simulink model "MPC_framework"  (Simulink 6.4)
settings: Solver=FixedStepDiscrete  StartTime=0.0  StopTime=10.0  FixedStep=0.01  RelTol=1e-3
PreLoadFcn:
  | RTWConfigurationCB('preloadfcn', bdroot);
InitFcn:
  | % START RTW CONFIGURATION CODE %
  | RTWConfigurationCB('rtw_target_initfcn',gcs);
  | % END RTW CONFIGURATION CODE %
undefined symbols (not defined in the file): a1, a2, DA_max_saturation, DA_min_saturation, DiscIntNeverNeededParam, fundamental_sample_time, incntr_half_val, init_1_message, init_2_message, init_ack_async_message, init_ack_sync_message, motor_negative_value_seg_1, motor_negative_value_seg_2, motor_positive_value_seg_1, motor_positive_value_seg_2, motor_stopped_value, ticks_per_trajectory_time, trajectory_time
libraries: canblocks x16, mpc555toucan x16, simulink x8, mpc555drivers x1
(part 2 of 2)

== stateflow chart State Machine ==
  settings: updateMethod=DISCRETE  sampleTime=0.01  executeAtInitialization=1
  state INIT
    entry: init_out_value=init_1_message;
    init_out_enable=1;
  state INIT_ACK
    entry: init_out_enable=0;
    init_out_value=init_2_message;
    init_out_trigger=1;
  state OPERATION
    entry: operation_mode=255;
    controller_enable=0;
    trajectory_enable=0;
    state PRIMITIVE
      entry: operation_mode=1;
      during: controller_enable=0;
      exit: motor1_reference=motor_stopped_value;
      motor2_reference=motor_stopped_value;
      state STOPPED
        entry: motor1_reference=motor_stopped_value;
        motor2_reference=motor_stopped_value;
        da_out_trigger=1;
        during: motor1_reference=motor_stopped_value;
        motor2_reference=motor_stopped_value;
        da_out_trigger=1;
        exit: stop_trigger=0;
      state MOVING
        state POSITIVE_MOV_SEG_1
          entry: motor2_reference=motor_stopped_value;
          during:
          motor1_reference=motor_positive_value_seg_1;
          da_out_trigger=1;
        state NEGATIVE_MOV_SEG_1
          entry: motor2_reference=motor_stopped_value;
          during:
          motor1_reference=motor_negative_value_seg_1;
          da_out_trigger=1;
        state POSITIVE_MOV_SEG_2
          entry: motor1_reference=motor_stopped_value;
          during:
          motor2_reference=motor_positive_value_seg_2;
          da_out_trigger=1;
        state NEGATIVE_MOV_SEG_2
          entry: motor1_reference=motor_stopped_value;
          during:
          motor2_reference=motor_negative_value_seg_2;
          da_out_trigger=1;
      (default) -> STOPPED
      MOVING -> STOPPED : [primitive_button==5]
      STOPPED -> POSITIVE_MOV_SEG_1 [order 4] : [primitive_button==1]
      STOPPED -> NEGATIVE_MOV_SEG_1 [order 2] : [primitive_button==3]
      STOPPED -> POSITIVE_MOV_SEG_2 [order 3] : [primitive_button==2]
      STOPPED -> NEGATIVE_MOV_SEG_2 [order 1] : [primitive_button==4]
    state CONTROLLER
      entry: operation_mode=2;
      alpha1_ref=alpha_in[0];
      alpha2_ref=alpha_in[1];
      motor1_reference=alpha1_ref;
      motor2_reference=alpha2_ref;
      trajectory_enable=0;
      controller_enable=1;
      da_out_trigger=1;
      exit: motor1_reference=motor_stopped_value;
      motor2_reference=motor_stopped_value;
      state HOLD
        entry:
        trajectory_ready=0;
        controller_message=4;
        send_controller_message;
        state HOLD_main
        state HOLD_wait
        (default) -> HOLD_main
        HOLD_main -> (junction 20) : [invgeo_done==1]
        (junction 21) -> HOLD_main : /send_controller_message
        (junction 20) -> (junction 23) [order 1] : [invgeo_error==0]{controller_message=1}
        (junction 20) -> (junction 24) [order 2] : [invgeo_error==1]{controller_message=2}
        (junction 20) -> HOLD_wait [order 3] : [invgeo_error>1]
        (junction 23) -> (junction 25) : /trajectory_ready=1
        (junction 24) -> (junction 26) : /trajectory_ready=0;
        (junction 25) -> (junction 27)
        (junction 26) -> (junction 27)
        (junction 27) -> (junction 21) : /invgeo_error=255
        HOLD_wait -> (junction 20) : [invgeo_error<2]
      state TRAJECTORY
        entry: controller_message=3;
        send_controller_message;
        trajectory_enable=1;
        exit:
        alpha1_ref=invgeo_alpha_1;
        alpha2_ref=invgeo_alpha_2;
        motor1_reference=alpha1_ref;
        motor2_reference=alpha2_ref;
        invgeo_error=255;
        trajectory_enable=0;
      TRAJECTORY -> HOLD : at(ticks_per_trajectory_time, tick)
      (junction 22) -> TRAJECTORY : [trajectory_ready==1]
      (default) -> HOLD
      HOLD -> (junction 22) : [async_request==9]
    state CONFIG
      entry: operation_mode=3;
      motor1_reference=motor_stopped_value;
      motor2_reference=motor_stopped_value;
      during: controller_enable=0;
      sync_command=0;
    state BLUETOOTH
      entry: operation_mode=4;
      motor1_reference=motor_stopped_value;
      motor2_reference=motor_stopped_value;
      during: controller_enable=0;
    (default) -> PRIMITIVE
    PRIMITIVE -> CONTROLLER [order 1] : [async_request==2]
    CONTROLLER -> PRIMITIVE [order 3] : [async_request==1]
    PRIMITIVE -> CONFIG [order 3] : [async_request==6]
    CONTROLLER -> CONFIG [order 2] : [async_request==6]
    CONFIG -> PRIMITIVE [order 1] : [async_request==1]
    CONFIG -> CONTROLLER [order 2] : [async_request==2]
    CONFIG -> CONFIG [order 7] : [async_request==3]{sync_command=1}
    CONFIG -> CONFIG [order 6] : [async_request==4]{sync_command=2}
    CONFIG -> CONFIG [order 5] : [async_request==5]{sync_command=3}
    CONFIG -> CONFIG [order 4] : [async_request==7]{sync_command=4}
    CONTROLLER -> BLUETOOTH [order 1] : [async_request==8]
    PRIMITIVE -> BLUETOOTH [order 2] : [async_request==8]
    CONFIG -> BLUETOOTH [order 3] : [async_request==8]
    BLUETOOTH -> CONFIG [order 3] : [async_request==6]
    BLUETOOTH -> CONTROLLER [order 2] : [async_request==2]
    BLUETOOTH -> PRIMITIVE [order 1] : [async_request==1]
  (default) -> INIT
  INIT -> INIT_ACK : [init_ack_sync==1 && init_ack_async==1]
  INIT_ACK -> OPERATION
  data: init_out_value output uint8 =0; init_out_enable output uint8 =0; init_ack_sync input uint8; init_ack_async input uint8; init_out_trigger output uint8 =0; stop_trigger output uint8 =0; primitive_button input uint8 =0; motor1_reference output single =hex2dec('8000'); motor2_reference output single =hex2dec('8000'); motor_stopped_value parameter uint16 =hex2dec('8000'); controller_enable output single =0; init_1_message parameter uint8 =init_1_message; init_2_message parameter uint8 =init_2_message; motor_positive_value_seg_1 parameter uint16; motor_negative_value_seg_1 parameter uint16; da_out_trigger output single =0; async_request input single; operation_mode output uint8 =255; sync_command output uint8 =0; alpha1_ref local single; alpha2_ref local single; alpha_in input single size=[1 2]; controller_message output uint8; invgeo_error data_store_memory double; invgeo_done input uint8; trajectory_enable output uint8 =0; trajectory_time parameter single; invgeo_alpha_1 data_store_memory double; invgeo_alpha_2 data_store_memory double; ticks_per_trajectory_time parameter single; motor_positive_value_seg_2 parameter uint16; motor_negative_value_seg_2 parameter uint16; trajectory_ready local uint8
  events: send_controller_message output FUNCTION_CALL_EVENT

== matlab function Inverse geometry/Subsystem/invgeo ==
  data: x input single; y input single; al1_c input single; al2_c input single; a1 input single; a2 input single; al1 output single; al2 output single; error output uint8
function [al1, al2, error] = invgeo(x, y, al1_c, al2_c, a1, a2)
    
    d = sqrt(x^2 + y^2);
    if (d > (a1 + a2)) | (d < (a1 - a2))
        al1 = al1_c;
        al2 = al2_c;
        error = uint8(1);
        return;
    end
    
    cos_al2 = (x^2 + y^2 - a1^2 - a2^2) / (2 * a1 * a2);
    D = a1 + a2 * cos_al2;
    
    sin_al1_p = (D * y + x * sqrt(x^2 + y^2 - D^2)) / (x^2 + y^2);
    sin_al1_n = (D * y - x * sqrt(x^2 + y^2 - D^2)) / (x^2 + y^2);
    
    cos_al1_p = (D * x + y * sqrt(x^2 + y^2 - D^2)) / (x^2 + y^2);
    cos_al1_n = (D * x - y * sqrt(x^2 + y^2 - D^2)) / (x^2 + y^2);
    
    al1_1 = atan2(sin_al1_p, cos_al1_n);
    
    al1_2 = atan2(sin_al1_n, cos_al1_p);
    
    al2_p = acos(cos_al2);
    al2_n = -al2_p; 
    
    cos_al1_al2_1 = (x - a1 * cos(al1_1)) / a2;
    sin_al1_al2_1 = (y - a1 * sin(al1_1)) / a2;
    al1_al2_1 = atan2(sin_al1_al2_1, cos_al1_al2_1);
    al2_1 = al1_al2_1 - al1_1;
    
    cos_al1_al2_2 = (x - a1 * cos(al1_2)) / a2;
    sin_al1_al2_2 = (y - a1 * sin(al1_2)) / a2;
    al1_al2_2 = atan2(sin_al1_al2_2, cos_al1_al2_2);
    al2_2 = al1_al2_2 - al1_2;
    
    if (abs(al1_c - al1_1) < abs(al1_c - al1_2))
        al1 = al1_1;
        al2 = al2_1;
    else
        al1 = al1_2;
        al2 = al2_2;
    end
    
    error = uint8(0);  
end

== matlab function Trajectory design/Trajectory design1/Curve calculation/Joint reference singal 1 ==
  data: a0 input double; a1 input double; a2 input double; a3 input double; a4 input double; a5 input double; t_sim input double; qa output double; qap output double; qapp output double; t_end input double
function [qa,qap,qapp] = fcn(a0,a1,a2,a3,a4,a5,t_sim,t_end)
% This block supports an embeddable subset of the MATLAB language.
% See the help menu for details. 
if (t_sim>=t_end) 
    t_sim = t_end;
end   
T = [t_sim^5/20 t_sim^4/12 t_sim^3/6 t_sim^2/2 t_sim 1;...
    t_sim^4/4 t_sim^3/3 t_sim^2/2 t_sim 1 0;...
    t_sim^3 t_sim^2 t_sim 1 0 0];
Q = T*[a0;a1;a2;a3;a4;a5];

qa = Q(1);
qap = Q(2);
qapp = Q(3);

== matlab function Trajectory design/Trajectory design1/Curve calculation/Joint reference singal 2 ==
  data: a0 input double; a1 input double; a2 input double; a3 input double; a4 input double; a5 input double; t_sim input double; qa output double; qap output double; qapp output double; t_end input double
function [qa,qap,qapp] = fcn(a0,a1,a2,a3,a4,a5,t_sim,t_end)
% This block supports an embeddable subset of the MATLAB language.
% See the help menu for details. 
if (t_sim>=t_end) 
    t_sim = t_end;
end   
T = [t_sim^5/20 t_sim^4/12 t_sim^3/6 t_sim^2/2 t_sim 1;...
    t_sim^4/4 t_sim^3/3 t_sim^2/2 t_sim 1 0;...
    t_sim^3 t_sim^2 t_sim 1 0 0];
Q = T*[a0;a1;a2;a3;a4;a5];

qa = Q(1);
qap = Q(2);
qapp = Q(3);

== matlab function Trajectory design/Trajectory design1/Init/Trajectory design 1 ==
  data: A input double; B input double; t input double; a0 output double; a1 output double; a2 output double; a3 output double; a4 output double; a5 output double
function [a0,a1,a2,a3,a4,a5] = fcn(A,B,t)
% This block supports an embeddable subset of the MATLAB language.
% See the help menu for details. 
T = [t^5/20 t^4/12 t^3/6 t^2/2 t 1;t^4/4 t^3/3 t^2/2 t 1 0;t^3 t^2 t 1 0 0;0 0 0 0 0 1;0 0 0 0 1 0;0 0 0 1 0 0];
Ao = inv(T)*[B;0;0;A;0;0];
a0=Ao(1);
a1=Ao(2);
a2=Ao(3);
a3=Ao(4);
a4=Ao(5);
a5=Ao(6);

== matlab function Trajectory design/Trajectory design1/Init/Trajectory design 2 ==
  data: A input double; B input double; t input double; a0 output double; a1 output double; a2 output double; a3 output double; a4 output double; a5 output double
function [a0,a1,a2,a3,a4,a5] = fcn(A,B,t)
% This block supports an embeddable subset of the MATLAB language.
% See the help menu for details. 
T = [t^5/20 t^4/12 t^3/6 t^2/2 t 1;t^4/4 t^3/3 t^2/2 t 1 0;t^3 t^2 t 1 0 0;0 0 0 0 0 1;0 0 0 0 1 0;0 0 0 1 0 0];
Ao = inv(T)*[B;0;0;A;0;0];
a0=Ao(1);
a1=Ao(2);
a2=Ao(3);
a3=Ao(4);
a4=Ao(5);
a5=Ao(6);
